simulink model "solar_collector_hot_water_storage"  (R2017a)
settings: Solver=VariableStepAuto  StartTime=0.0  StopTime=100000  RelTol=1e-3
values from neighbouring files (symbols this model uses):
  a1 = Ac*eta/C_c    (= 0.000575964912281)    [Linearized_model.m]    (also in Linearized_model_v1.m; Maple_linearization.m = 0.000380952380952; solar_collector_init.m = 7.33988724098e-05)
  a2 = -U_L1*Ac/2/C_c    (= -0.00145487240829)    [Linearized_model.m]    (also in Linearized_model_v1.m = -0.00290974481659; Maple_linearization.m = 0.00111111111111; solar_collector_init.m = -0.000214080044529)
  a3 = -U_L2*Ac/C_c    (= -7.48006379585e-06)    [Linearized_model.m]    (also in Linearized_model_v1.m; Maple_linearization.m = -0.00222222222222; solar_collector_init.m = 0.000428160089057)
  a4 = V_c^-1    (= 333.333333333)    [Linearized_model.m]    (also in Linearized_model_v1.m; Maple_linearization.m = 666.666666667; solar_collector_init.m = 133.333333333)
  a5 = -a4    (= -333.333333333)    [Linearized_model.m]    (also in Linearized_model_v1.m; Maple_linearization.m = -666.666666667; solar_collector_init.m = -133.333333333)
libraries: simulink x2
settings Model: Creator=info  LastModifiedBy=admin

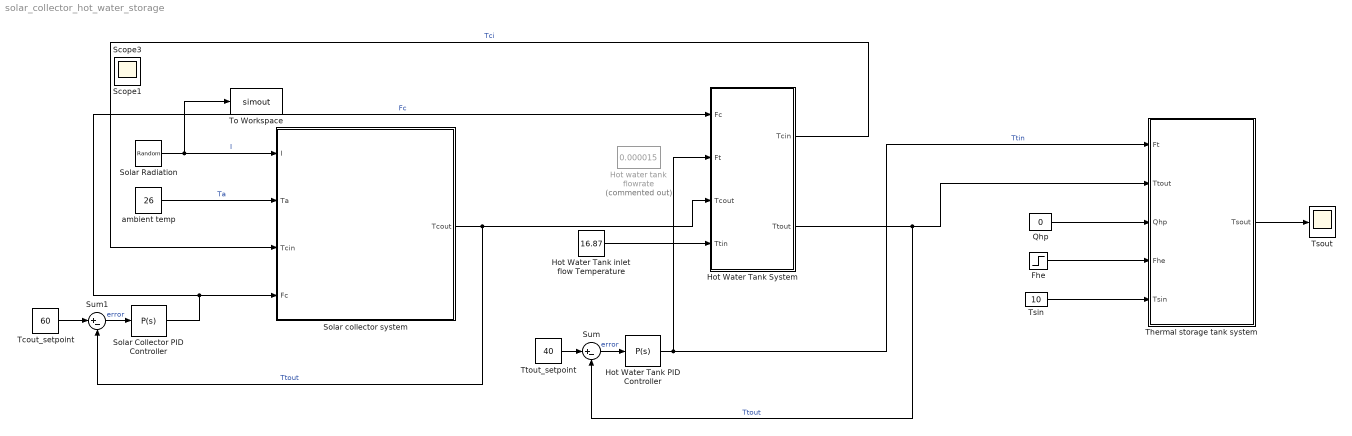
== system solar_collector_hot_water_storage ==
  "Fhe " : Step  Time=5  After=0.000015  SampleTime=0
  Hot Water Tank PID Controller : simulink/Continuous/PID Controller  Controller=P  TimeDomain=Continuous-time  SampleTime=-1  IntegratorMethod=Forward Euler  FilterMethod=Forward Euler  Form=Parallel  UseFilter=on  ControllerParametersSource=internal  P=-0.0002  I=1.2  D=0.01  N=100  InitialConditionSource=internal  InitialConditionForIntegrator=0  InitialConditionForFilter=0  ExternalReset=none  ZeroCross=off  LimitOutput=on  UpperSaturationLimit=0.00015  LowerSaturationLimit=0  LinearizeAsGain=on  AntiWindupMode=none  Kb=1  TrackingMode=off  Kt=1  PParamMin=[]  PParamMax=[]  IParamMin=[]  IParamMax=[]  DParamMin=[]  DParamMax=[]  NParamMin=[]  NParamMax=[]  KbParamMin=[]  KbParamMax=[]  KtParamMin=[]  KtParamMax=[]  POutMin=[]  POutMax=[]  IOutMin=[]  IOutMax=[]  DOutMin=[]  DOutMax=[]  NOutMin=[]  NOutMax=[]  KbOutMin=[]  KbOutMax=[]  KtOutMin=[]  KtOutMax=[]  IntegratorOutMin=[]  IntegratorOutMax=[]  FilterOutMin=[]  FilterOutMax=[]  SumOutMin=[]  SumOutMax=[]  SumI1OutMin=[]  SumI1OutMax=[]  SumI2OutMin=[]  SumI2OutMax=[]  SumI3OutMin=[]  SumI3OutMax=[]  SumDOutMin=[]  SumDOutMax=[]  SaturationOutMin=[]  SaturationOutMax=[]  IntegratorContinuousStateAttributes=''  IntegratorStateMustResolveToSignalObject=off  IntegratorRTWStateStorageClass=Auto  FilterContinuousStateAttributes=''  FilterStateMustResolveToSignalObject=off  FilterRTWStateStorageClass=Auto  DifferentiatorICPrevScaledInput=0  DifferentiatorOutMin=[]  DifferentiatorOutMax=[]  InitialConditionSetting=State (most efficient)
  Hot Water Tank System : Subsystem
      mask Display: image('hot_water_tank.PNG');
  Hot Water Tank inlet flow Temperature : Constant  Value=16.87
  Hot water tank flowrate : Constant  Commented=on  Value=0.000015
  Qhp : Constant  Value=0
  Solar Collector PID Controller : simulink/Continuous/PID Controller  Controller=P  TimeDomain=Continuous-time  SampleTime=-1  IntegratorMethod=Forward Euler  FilterMethod=Forward Euler  Form=Parallel  UseFilter=on  ControllerParametersSource=internal  P=-0.0002  I=1.2  D=0.01  N=100  InitialConditionSource=internal  InitialConditionForIntegrator=0  InitialConditionForFilter=0  ExternalReset=none  ZeroCross=off  LimitOutput=on  UpperSaturationLimit=0.00015  LowerSaturationLimit=0  LinearizeAsGain=on  AntiWindupMode=none  Kb=1  TrackingMode=off  Kt=1  PParamMin=[]  PParamMax=[]  IParamMin=[]  IParamMax=[]  DParamMin=[]  DParamMax=[]  NParamMin=[]  NParamMax=[]  KbParamMin=[]  KbParamMax=[]  KtParamMin=[]  KtParamMax=[]  POutMin=[]  POutMax=[]  IOutMin=[]  IOutMax=[]  DOutMin=[]  DOutMax=[]  NOutMin=[]  NOutMax=[]  KbOutMin=[]  KbOutMax=[]  KtOutMin=[]  KtOutMax=[]  IntegratorOutMin=[]  IntegratorOutMax=[]  FilterOutMin=[]  FilterOutMax=[]  SumOutMin=[]  SumOutMax=[]  SumI1OutMin=[]  SumI1OutMax=[]  SumI2OutMin=[]  SumI2OutMax=[]  SumI3OutMin=[]  SumI3OutMax=[]  SumDOutMin=[]  SumDOutMax=[]  SaturationOutMin=[]  SaturationOutMax=[]  IntegratorContinuousStateAttributes=''  IntegratorStateMustResolveToSignalObject=off  IntegratorRTWStateStorageClass=Auto  FilterContinuousStateAttributes=''  FilterStateMustResolveToSignalObject=off  FilterRTWStateStorageClass=Auto  DifferentiatorICPrevScaledInput=0  DifferentiatorOutMin=[]  DifferentiatorOutMax=[]  InitialConditionSetting=State (most efficient)
  Solar Radiation : RandomNumber  Mean=1360  Variance=0.5  SampleTime=0.1
  Solar collector system : Subsystem
      mask Display: image('collector_image.jpg');
  Sum : Sum  Inputs=|+-
  Sum1 : Sum  Inputs=|+-
  Tcout_setpoint : Constant  Value=60
  Thermal storage tank system : Subsystem
      mask Display: image('storage_tank.PNG');
  To Workspace : ToWorkspace  VariableName=simout  SaveFormat=Timeseries  SampleTime=-1
  Tsin : Constant  Value=10
  Tsout : Scope
  Ttout_setpoint : Constant  Value=40
  ambient temp : Constant  Value=26
  Scope1 : Scope
  Scope3 : Scope
  wires:
  Hot Water Tank System/1("Tcin ") -> Solar collector system/3(Tcin)  "Tci"
  ambient temp/1 -> Solar collector system/2(Ta)  "Ta"
  Solar Radiation/1 -> To Workspace/1, Solar collector system/1(I)  "I"
  Hot Water Tank System/2("Ttout ") -> Thermal storage tank system/2("Ttout "), Sum/2  "Ttout"
  Ttout_setpoint/1 -> Sum/1
  Sum/1 -> Hot Water Tank PID Controller/1  "error"
  Solar Collector PID Controller/1 -> Hot Water Tank System/1("Fc "), Solar collector system/4(Fc)  "Fc"
  Hot Water Tank PID Controller/1 -> Thermal storage tank system/1("Ft "), Hot Water Tank System/2(Ft)  "Ttin"
  Hot Water Tank inlet flow Temperature/1 -> Hot Water Tank System/4("Ttin ")
  Sum1/1 -> Solar Collector PID Controller/1  "error"
  Tcout_setpoint/1 -> Sum1/1
  Solar collector system/1(Tcout) -> Sum1/2, Hot Water Tank System/3("Tcout ")  "Ttout"
  Qhp/1 -> Thermal storage tank system/3(Qhp)
  Thermal storage tank system/1("Tsout ") -> Tsout/1
  "Fhe "/1 -> Thermal storage tank system/4(Fhe)
  Tsin/1 -> Thermal storage tank system/5(Tsin)

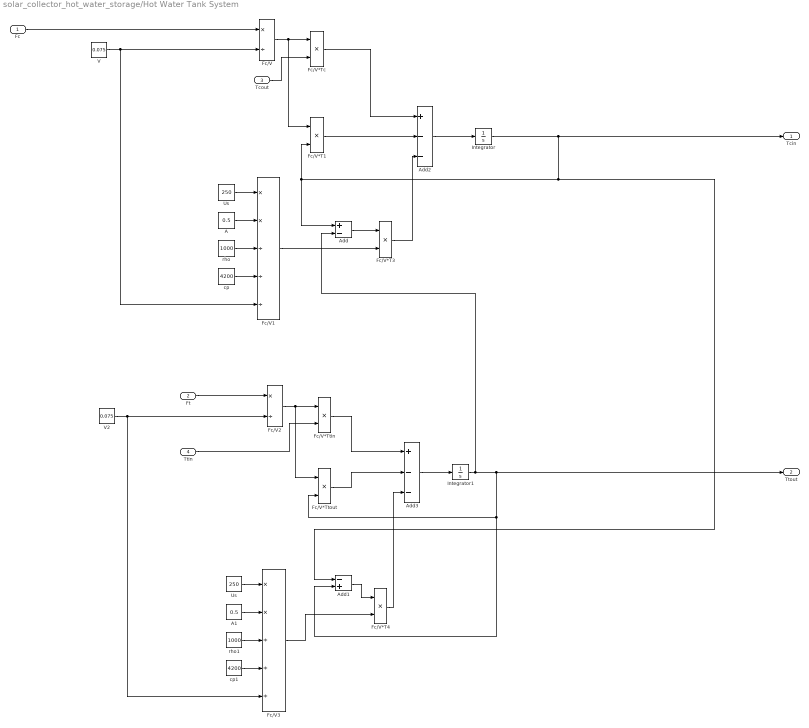
== system solar_collector_hot_water_storage/Hot Water Tank System ==
  "Fc " : Inport
  Ft : Inport  Port=2
  "Tcout " : Inport  Port=3
  "Ttin " : Inport  Port=4
  A : Constant  Value=0.5
  A1 : Constant  Value=0.5
  Add : Sum  Inputs=+-
  Add1 : Sum  Inputs=-+
  Add2 : Sum  Inputs=+--
  Add3 : Sum  Inputs=+--
  Fc/V : Product  Inputs=*/
  Fc/V*T1 : Product  Inputs=**
  Fc/V*T3 : Product  Inputs=**
  Fc/V*T4 : Product  Inputs=**
  Fc/V*Tc : Product  Inputs=**
  Fc/V*Ttin : Product  Inputs=**
  Fc/V*Ttout : Product  Inputs=**
  Fc/V1 : Product  Inputs=**///
  Fc/V2 : Product  Inputs=*/
  Fc/V3 : Product  Inputs=**///
  Integrator : Integrator  InitialCondition=16.87
  Integrator1 : Integrator  InitialCondition=10
  Us : Constant  Value=250
  "Us    " : Constant  Value=250
  V : Constant  Value=0.075
  V2 : Constant  Value=0.075
  cp : Constant  Value=4200
  cp1 : Constant  Value=4200
  rho : Constant  Value=1000
  rho1 : Constant  Value=1000
  "Tcin " : Outport
  "Ttout " : Outport  Port=2
  wires:
  V/1 -> Fc/V1/5, Fc/V/2
  "Us    "/1 -> Fc/V3/1
  Integrator1/1 -> Add1/2, Fc/V*Ttout/2, "Ttout "/1, Add/2
  "Ttin "/1 -> Fc/V*Ttin/2
  "Fc "/1 -> Fc/V/1
  Fc/V/1 -> Fc/V*T1/1, Fc/V*Tc/1
  rho/1 -> Fc/V1/3
  cp1/1 -> Fc/V3/4
  A1/1 -> Fc/V3/2
  Integrator/1 -> "Tcin "/1, Add1/1, Fc/V*T1/2, Add/1
  Us/1 -> Fc/V1/1
  "Tcout "/1 -> Fc/V*Tc/2
  rho1/1 -> Fc/V3/3
  Fc/V2/1 -> Fc/V*Ttin/1, Fc/V*Ttout/1
  V2/1 -> Fc/V2/2, Fc/V3/5
  Ft/1 -> Fc/V2/1
  cp/1 -> Fc/V1/4
  A/1 -> Fc/V1/2
  Fc/V*Tc/1 -> Add2/1
  Add2/1 -> Integrator/1
  Fc/V1/1 -> Fc/V*T3/2
  Fc/V*T3/1 -> Add2/3
  Fc/V*Ttin/1 -> Add3/1
  Add3/1 -> Integrator1/1
  Add/1 -> Fc/V*T3/1
  Fc/V*T1/1 -> Add2/2
  Fc/V*Ttout/1 -> Add3/2
  Fc/V*T4/1 -> Add3/3
  Fc/V3/1 -> Fc/V*T4/2
  Add1/1 -> Fc/V*T4/1

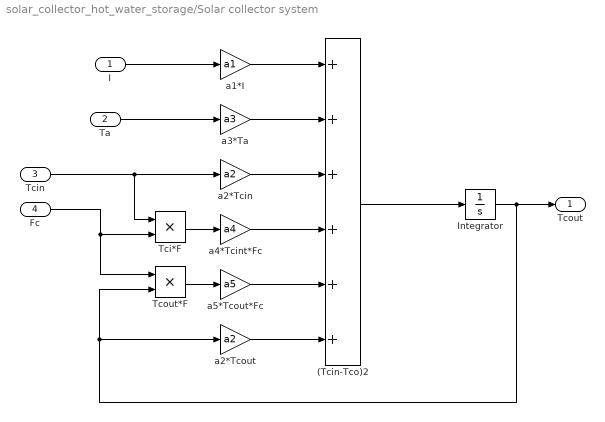
== system solar_collector_hot_water_storage/Solar collector system ==
  I : Inport
  Ta : Inport  Port=2
  Tcin : Inport  Port=3
  Fc : Inport  Port=4
  (Tcin-Tco)2 : Sum  Inputs=++++++
  Integrator : Integrator  InitialCondition=10
  Tci*F : Product  Inputs=**
  Tcout*F : Product  Inputs=**
  a1*I : Gain  Gain=a1
  a2*Tcin : Gain  Gain=a2
  "a2*Tcout " : Gain  Gain=a2
  a3*Ta : Gain  Gain=a3
  a4*Tcint*Fc : Gain  Gain=a4
  "a5*Tcout*Fc " : Gain  Gain=a5
  Tcout : Outport
  wires:
  I/1 -> a1*I/1
  Integrator/1 -> "a2*Tcout "/1, Tcout*F/2, Tcout/1
  (Tcin-Tco)2/1 -> Integrator/1
  Fc/1 -> Tcout*F/1, Tci*F/2
  a1*I/1 -> (Tcin-Tco)2/1
  Ta/1 -> a3*Ta/1
  Tcin/1 -> Tci*F/1, a2*Tcin/1
  a3*Ta/1 -> (Tcin-Tco)2/2
  a2*Tcin/1 -> (Tcin-Tco)2/3
  "a5*Tcout*Fc "/1 -> (Tcin-Tco)2/5
  Tci*F/1 -> a4*Tcint*Fc/1
  a4*Tcint*Fc/1 -> (Tcin-Tco)2/4
  Tcout*F/1 -> "a5*Tcout*Fc "/1
  "a2*Tcout "/1 -> (Tcin-Tco)2/6

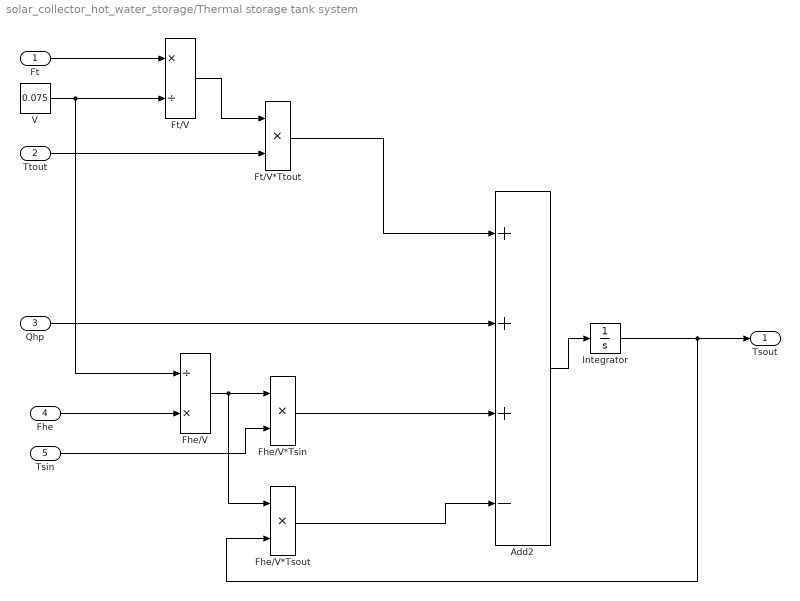
== system solar_collector_hot_water_storage/Thermal storage tank system ==
  "Ft " : Inport
  "Ttout " : Inport  Port=2
  Qhp : Inport  Port=3
  Fhe : Inport  Port=4
  Tsin : Inport  Port=5
  Add2 : Sum  Inputs=+++-
  Fhe/V : Product  Inputs=/*
  Fhe/V*Tsin : Product  Inputs=**
  Fhe/V*Tsout : Product  Inputs=**
  Ft/V : Product  Inputs=*/
  Ft/V*Ttout : Product  Inputs=**
  Integrator : Integrator  InitialCondition=16.87
  V : Constant  Value=0.075
  "Tsout " : Outport
  wires:
  "Ft "/1 -> Ft/V/1
  Ft/V/1 -> Ft/V*Ttout/1
  Integrator/1 -> "Tsout "/1, Fhe/V*Tsout/2
  "Ttout "/1 -> Ft/V*Ttout/2
  Ft/V*Ttout/1 -> Add2/1
  Add2/1 -> Integrator/1
  Tsin/1 -> Fhe/V*Tsin/2
  Fhe/V/1 -> Fhe/V*Tsout/1, Fhe/V*Tsin/1
  Fhe/V*Tsin/1 -> Add2/3
  V/1 -> Fhe/V/1, Ft/V/2
  Fhe/1 -> Fhe/V/2
  Qhp/1 -> Add2/2
  Fhe/V*Tsout/1 -> Add2/4
